simulink model "Model_SIMEX"  (R2018a)
settings: Solver=VariableStepAuto  StartTime=0.0  StopTime=65  RelTol=1e-3
settings Model: Creator=Marco Passarella  LastModifiedBy=Marco Passarella

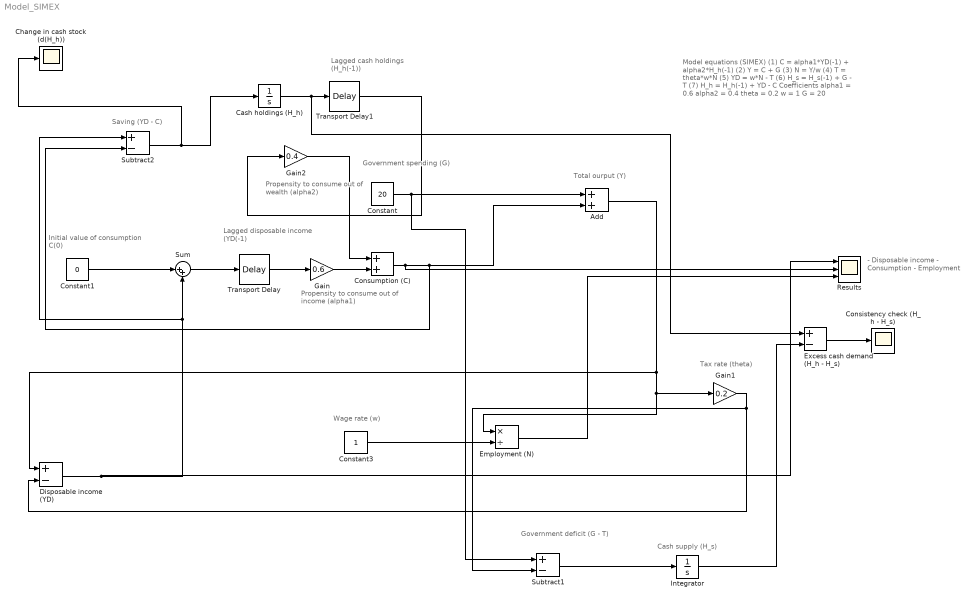
== system Model_SIMEX ==
  note: - Disposable income
      | - Consumption
      | - Employment
  note: Lagged cash
      | holdings (H_h(-1))
  note: Saving (YD - C)
  note: Cash supply (H_s)
  note: Government
      | deficit (G - T)
  note: Tax rate (theta)
  note: Wage rate (w)
  note: Lagged disposable
      | income (YD(-1)
  note: Initial value of
      | consumption C(0)
  note: Propensity to
      | consume out
      | of income (alpha1)
  note: Total ourput (Y)
  note: Government
      | spending (G)
  note: Model equations (SIMEX)
      | (1) C = alpha1*YD(-1) + alpha2*H_h(-1)
      | (2) Y = C + G
      | (3) N = Y/w
      | (4) T = theta*w*N
      | (5) YD = w*N - T
      | (6) H_s = H_s(-1) + G - T
      | (7) H_h = H_h(-1) + YD - C
      |
      | Coefficients
      | alpha1 = 0.6
      | alpha2 = 0.4
      | theta = 0.2
      | w = 1
      | G = 20
  note: Propensity to
      | consume out
      | of wealth (alpha2)
  Add : Sum
  Cash holdings (H_h) : Integrator
  Change in cash stock (d(H_h)) : Scope
  Consistency check (H_h - H_s) : Scope
  Constant : Constant  Value=20
  Constant1 : Constant  Value=0
  Constant3 : Constant
  Consumption (C) : Sum
  Disposable income (YD) : Sum  Inputs=+-
  Employment (N) : Product  Inputs=*/
  Excess cash demand (H_h - H_s) : Sum  Inputs=+-
  Gain : Gain  Gain=0.6
  Gain1 : Gain  Gain=0.2
  Gain2 : Gain  Gain=0.4
  Integrator : Integrator
  Results : Scope  NumInputPorts=3
  Subtract1 : Sum  Inputs=+-
  Subtract2 : Sum  Inputs=+-
  Sum : Sum  Inputs=|++
  Transport Delay : TransportDelay
  Transport Delay1 : TransportDelay
  wires:
  Constant/1 -> Subtract1/1, Add/1
  Add/1 -> Disposable income (YD)/1, Employment (N)/1, Gain1/1
  Consumption (C)/1 -> Results/2, Add/2, Subtract2/2
  Sum/1 -> Transport Delay/1
  Transport Delay/1 -> Gain/1
  Gain/1 -> Consumption (C)/2
  Constant1/1 -> Sum/1
  Constant3/1 -> Employment (N)/2
  Gain1/1 -> Subtract1/2, Disposable income (YD)/2
  Disposable income (YD)/1 -> Results/1, Subtract2/1, Sum/2
  Subtract1/1 -> Integrator/1
  Subtract2/1 -> Change in cash stock (d(H_h))/1, Cash holdings (H_h)/1
  Cash holdings (H_h)/1 -> Excess cash demand (H_h - H_s)/1, Transport Delay1/1
  Transport Delay1/1 -> Gain2/1
  Gain2/1 -> Consumption (C)/1
  Integrator/1 -> Excess cash demand (H_h - H_s)/2
  Employment (N)/1 -> Results/3
  Excess cash demand (H_h - H_s)/1 -> Consistency check (H_h - H_s)/1
